simulink model "piv_simulation"  (R2022b)
settings: Solver=FixedStepAuto  StartTime=0.0  StopTime=40  FixedStep=0.01  RelTol=1e-3
values from neighbouring files (symbols this model uses):
  AW = 5    [pos_piv.m]
  I = 3.5926734620137482    (= 3.59267346201)    [pos_piv.m]
  P = 1.0526315789473684    (= 1.05263157895)    [pos_piv.m]
  Ts = 0.01    [pos_piv.m]
  u_max = 100    [pos_piv.m]
  u_min = -100    [pos_piv.m]
  V = 0.76904319363933893    (= 0.769043193639)    [pos_piv.m]
libraries: cstblocks x3
settings Model: Creator=ladislav  LastModifiedBy=ladislav

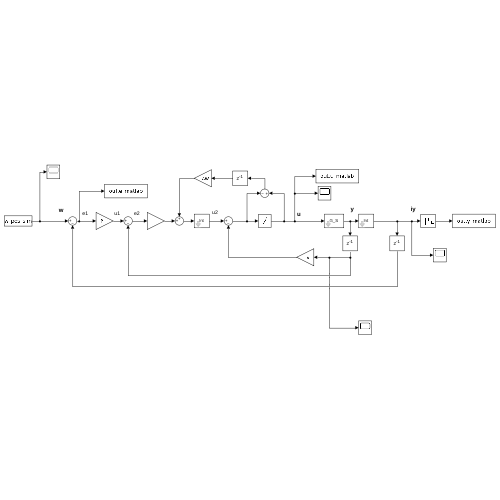
[thumbnail: Simulink's stored preview of the top-level diagram]
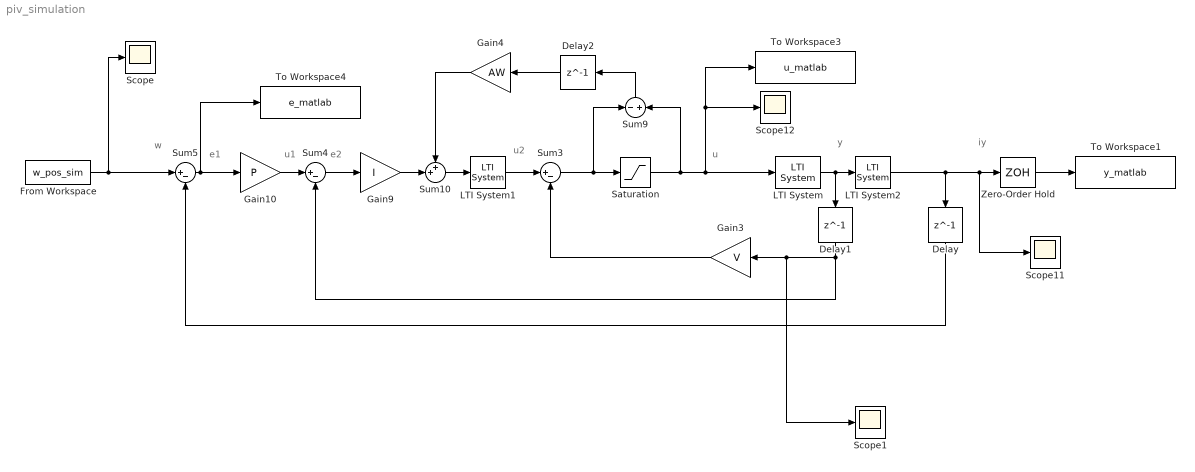
== system piv_simulation ==
  note: w
  note: iy
  note: u
  note: u2
  note: e1
  note: e2
  note: u1
  note: y
  Delay : Delay  DelayLength=1
  Delay1 : Delay  DelayLength=1
  Delay2 : Delay  DelayLength=1
  From Workspace : FromWorkspace  VariableName=w_pos_sim  SampleTime=Ts
  Gain10 : Gain  Gain=P
  Gain3 : Gain  Gain=V
  Gain4 : Gain  Gain=AW
  Gain9 : Gain  Gain=I
  LTI System : cstblocks/LTI System  sys=G_S  IC=[]
  LTI System1 : cstblocks/LTI System  sys=Int  IC=[]
  LTI System2 : cstblocks/LTI System  sys=Int  IC=[]
  Saturation : Saturate  UpperLimit=u_max  LowerLimit=u_min  LinearizeAsGain=off
  Scope{,1,11..12} (4 alike) : Scope
  Sum10 : Sum  Inputs=++|
  Sum3 : Sum  Inputs=|+-
  Sum4 : Sum  Inputs=|+-
  Sum5 : Sum  Inputs=|+-
  Sum9 : Sum  Inputs=-|+
  To Workspace1 : ToWorkspace  VariableName=y_matlab  SaveFormat=Timeseries  SampleTime=-1
  To Workspace3 : ToWorkspace  VariableName=u_matlab  SaveFormat=Timeseries  SampleTime=-1
  To Workspace4 : ToWorkspace  VariableName=e_matlab  SaveFormat=Timeseries  SampleTime=-1
  Zero-Order Hold : ZeroOrderHold  SampleTime=0.01
  wires:
  Sum5/1 -> To Workspace4/1, Gain10/1
  Gain3/1 -> Sum3/2
  LTI System/1 -> LTI System2/1, Delay1/1
  LTI System1/1 -> Sum3/1
  Sum3/1 -> Sum9/1, Saturation/1
  Gain10/1 -> Sum4/1
  From Workspace/1 -> Sum5/1, Scope/1
  LTI System2/1 -> Scope11/1, Zero-Order Hold/1, Delay/1
  Sum4/1 -> Gain9/1
  Sum10/1 -> LTI System1/1
  Gain9/1 -> Sum10/2
  Sum9/1 -> Delay2/1
  Delay/1 -> Sum5/2
  Delay1/1 -> Scope1/1, Gain3/1, Sum4/2
  Gain4/1 -> Sum10/1
  Delay2/1 -> Gain4/1
  Saturation/1 -> Sum9/2, LTI System/1, Scope12/1, To Workspace3/1
  Zero-Order Hold/1 -> To Workspace1/1
